simulink model "VSI_o_loop_Gvd"  (Simulink 7.8)
settings: Solver=ode23t  StartTime=0.0  StopTime=0.5  MaxStep=25e-6  RelTol=1e-4  AbsTol=1e-5
values from neighbouring files (symbols this model uses):
  C = 21.308e-6    (= 2.1308e-05)    [Current_Loop_Design.m]    (also in VSI_Controller_Design.m = 3.13e-05; VSI_TFs_i_loop.m = 2.2e-05; VSI_TFs_o_loop.m = 4.13e-05; VSI_TFs_v_loop.m = 4.1308e-05)
  Dd = -(omega*L*Voq-Rac*Vod-Rl*Vod+Rl*omega*C*Voq*Rac+omega^2*L*C*Vod*Rac)/(Rac*Vdc)    [Current_Loop_Design.m]    (also in ZVSI_il_tf_cal_sim_comp_frd_model_v1.m = Dd(length(Dd)-10); ZVSI_ol_tf_cal_sim_comp_frd_model_v1.m = 0.295957004555; ZVSI_vil_tf_cal_frd_model_Monte_Carlo.m; ZVSI_vil_tf_cal_sim_comp_frd_model_v1.m = Dd(length(Dd)-10))
  Dq = -(-Rl*Voq-Rac*Voq-omega*L*Vod+omega^2*L*C*Voq*Rac-Rl*omega*C*Vod*Rac)/(Rac*Vdc)    [Current_Loop_Design.m]    (also in ZVSI_il_tf_cal_sim_comp_frd_model_v1.m = Dq(length(Dq)-10); ZVSI_ol_tf_cal_sim_comp_frd_model_v1.m = 0.0618083618596; ZVSI_vil_tf_cal_frd_model_Monte_Carlo.m; ZVSI_vil_tf_cal_sim_comp_frd_model_v1.m = Dq(length(Dq)-10))
  L = (0.75879e-3)/(2/3)    (= 0.001138185)    [Current_Loop_Design.m]    (also in VSI_Controller_Design.m = 0.0011; VSI_TFs_i_loop.m = 0.0012; VSI_TFs_o_loop.m = 0.0011; VSI_TFs_v_loop.m = 0.0011)
  RL = 80e-3    (= 0.08)    [Current_Loop_Design.m]    (also in ZVSI_il_tf_cal_sim_comp_frd_model_v1.m = 0.15; ZVSI_ol_tf_cal_sim_comp_frd_model_v1.m = 1.5e-05; ZVSI_vil_tf_cal_frd_model_Monte_Carlo.m = 0.13; ZVSI_vil_tf_cal_sim_comp_frd_model_v1.m = 0.13)
  Vdc = 270    [Current_Loop_Design.m]    (also in VSI_Controller_Design.m; VSI_TFs_i_loop.m; VSI_TFs_o_loop.m; VSI_TFs_v_loop.m)
  w = 2*pi*fline    (= 2513.27412287)    [Current_Loop_Design.m]    (also in ZVSI_il_tf_cal_sim_comp_frd_model_v1.m = 15791.3670417; ZVSI_ol_tf_cal_sim_comp_frd_model_v1.m = 15791.3670417; ZVSI_vil_tf_cal_frd_model_Monte_Carlo.m = 15791.3670417; ZVSI_vil_tf_cal_sim_comp_frd_model_v1.m = 15791.3670417)
libraries: powerlib x20
settings Model: Creator=marko  LastModifiedBy=wenbo  BufferReuse=off
settings OptimizationCC: BlockReduction=off  InlineParams=on  BufferReuse=off
settings DebuggingCC: AlgebraicLoopMsg=none  SolverPrmCheckMsg=none  FcnCallInpInsideContextMsg=Use local settings  UnconnectedInputMsg=none  UnconnectedOutputMsg=none  UnconnectedLineMsg=none  StrictBusMsg=Warning

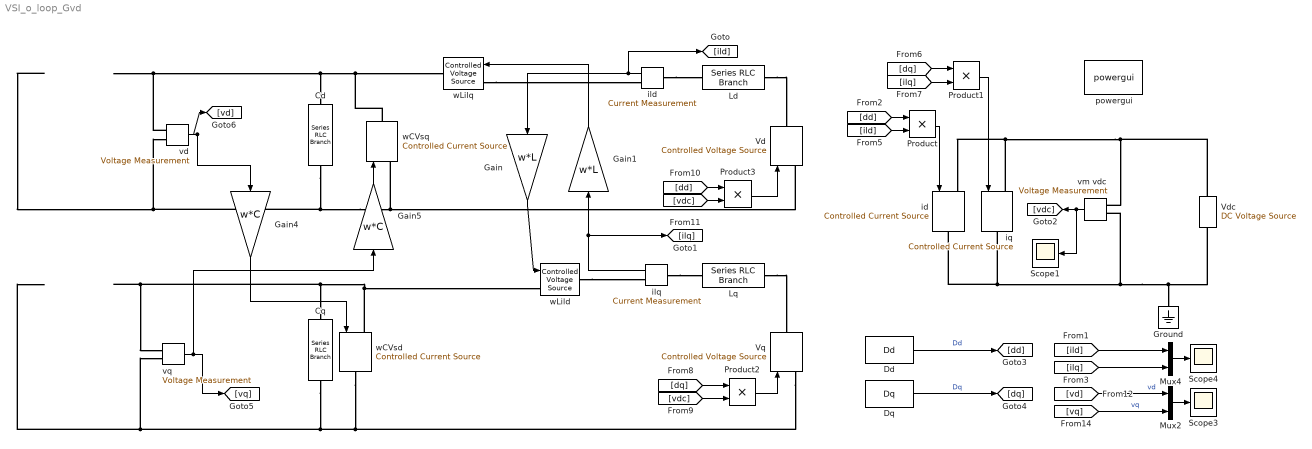
== system VSI_o_loop_Gvd ==
  Cd : powerlib/Elements/Series RLC Branch  LConnTagsString=__new0  RConnTagsString=__new0  BranchType=C  Resistance=1  Inductance=1e-3  SetiL0=off  InitialCurrent=0  Capacitance=C  Setx0=off  InitialVoltage=0  Measurements=None
  Cq : powerlib/Elements/Series RLC Branch  LConnTagsString=__new0  RConnTagsString=__new0  BranchType=C  Resistance=1  Inductance=1e-3  SetiL0=off  InitialCurrent=0  Capacitance=C  Setx0=off  InitialVoltage=0  Measurements=None
  Dd : Constant  Value=Dd
  Dq : Constant  Value=Dq
  Gain : Gain  Gain=w*L
  Gain1 : Gain  Gain=w*L
  Gain4 : Gain  Gain=w*C
  Gain5 : Gain  Gain=w*C
  Ground : powerlib/Elements/Ground  LConnTagsString=a
  Ld : powerlib/Elements/Series RLC Branch  LConnTagsString=__new0  RConnTagsString=__new0  BranchType=RL  Resistance=RL  Inductance=L  SetiL0=off  InitialCurrent=0  Capacitance=1e-6  Setx0=off  InitialVoltage=0  Measurements=None
  Lq : powerlib/Elements/Series RLC Branch  LConnTagsString=__new0  RConnTagsString=__new0  BranchType=RL  Resistance=RL  Inductance=L  SetiL0=off  InitialCurrent=0  Capacitance=1e-6  Setx0=off  InitialVoltage=0  Measurements=None
  Mux2 : Mux  Inputs=2
  Mux4 : Mux  Inputs=2
  Product{,1..3} (4 alike) : Product  RndMeth=Zero
  Scope1 : Scope
      settings: YMin=270  YMax=270  SaveName=ildq_matlab  DataFormat=Array
  Scope3 : Scope
      settings: YMin=-0.25  YMax=5.25  SaveName=ildq_matlab2  DataFormat=Array
  Scope4 : Scope
      settings: YMin=-0.25  YMax=5.25  SaveName=ildq_matlab1  DataFormat=Array
  Vd : powerlib/Electrical Sources/Controlled Voltage Source  Initialize=on  Source_Type=DC  Amplitude=0  Phase=0  Frequency=0  Measurements=None
  Vdc : powerlib/Electrical Sources/DC Voltage Source  Amplitude=Vdc  Measurements=None
  Vq : powerlib/Electrical Sources/Controlled Voltage Source  Initialize=on  Source_Type=DC  Amplitude=0  Phase=0  Frequency=0  Measurements=None
  id : powerlib/Electrical Sources/Controlled Current Source  Initialize=on  Source_Type=DC  Amplitude=0  Phase=0  Frequency=0  Measurements=None
  ild : powerlib/Measurements/Current Measurement  PhasorSimulation=off  OutputType=Complex  PSBequivalent=0
  ilq : powerlib/Measurements/Current Measurement  PhasorSimulation=off  OutputType=Complex  PSBequivalent=0
  iq : powerlib/Electrical Sources/Controlled Current Source  Initialize=on  Source_Type=DC  Amplitude=0  Phase=0  Frequency=0  Measurements=None
  powergui : powerlib/powergui  Priority=1  SimulationMode=Continuous  SolverType=Tustin  SampleTime=50e-6  frequency=60  SPID=off  DisableSnubberDevices=off  DisableRonSwitches=off  DisableVfSwitches=off  SwTol=0  Interpol=off  DisplayEquations=off  FunctionMessages=off  frequencyindice=0  Pbase=100e6  ErrMax=1e-4  Iterations=50  UnitsV=kV  UnitsW=MW  echomessages=off  HookPort=off  EnableUseOfTLC=off  x0status=blocks  RestoreLinks=warning  ResistiveCurrentMeasurement=off  Frange=[0:2:500]  Ylog=off  Xlog=on  ShowGrid=off  save=off  variable=ZData  ZoomFFT=on  StartTime=0.0  cycles=1  DisplayStyle=1  fundamental=60  FreqAxis=off  MaxFrequency=1000  frequencyindicesteady=1  RmsSteady=1  display=off  Ts=0  methode=off
  vd : powerlib/Measurements/Voltage Measurement  PhasorSimulation=off  OutputType=Complex  PSBequivalent=0
  vm vdc : powerlib/Measurements/Voltage Measurement  PhasorSimulation=off  OutputType=Complex  PSBequivalent=0
  vq : powerlib/Measurements/Voltage Measurement  PhasorSimulation=off  OutputType=Complex  PSBequivalent=0
  wCVsd : powerlib/Electrical Sources/Controlled Current Source  Initialize=on  Source_Type=DC  Amplitude=0  Phase=0  Frequency=0  Measurements=None
  wCVsq : powerlib/Electrical Sources/Controlled Current Source  Initialize=on  Source_Type=DC  Amplitude=0  Phase=0  Frequency=0  Measurements=None
  wLild : powerlib/Electrical Sources/Controlled Voltage Source  Initialize=on  Source_Type=DC  Amplitude=0  Phase=0  Frequency=0  Measurements=None
  wLilq : powerlib/Electrical Sources/Controlled Voltage Source  Initialize=on  Source_Type=DC  Amplitude=0  Phase=0  Frequency=0  Measurements=None
  wires:
  Product/1 -> id/1
  [dd] -> Product/1
  [ild] -> Product/2
  Product1/1 -> iq/1
  [dq] -> Product1/1
  [ilq] -> Product1/2
  [dq] -> Product2/1
  [vdc] -> Product2/2
  Product2/1 -> Vq/1
  [dd] -> Product3/1
  [vdc] -> Product3/2
  Product3/1 -> Vd/1
  vd/1 -> Gain4/1, [vd]
  vq/1 -> Gain5/1, [vq]
  vm vdc/1 -> [vdc], Scope1/1
  ilq/1 -> Gain1/1, [ilq]
  Gain1/1 -> wLilq/1
  ild/1 -> Gain/1, [ild]
  Gain/1 -> wLild/1
  Gain4/1 -> wCVsd/1
  Gain5/1 -> wCVsq/1
  Dd/1 -> [dd]  "Dd"
  Dq/1 -> [dq]  "Dq"
  [ild] -> Mux4/1
  [ilq] -> Mux4/2
  Mux4/1 -> Scope4/1
  [vd] -> Mux2/1  "vd"
  [vq] -> Mux2/2  "vq"
  Mux2/1 -> Scope3/1
  connections:
  Vq/LConn1 -- wCVsd/RConn1 -- Cq/RConn1 -- vq/LConn2
  iq/RConn1 -- id/RConn1 -- vm vdc/LConn2 -- Ground/LConn1 -- Vdc/LConn1
  Cq/LConn1 -- wCVsd/LConn1 -- wLild/LConn1 -- vq/LConn1
  wLilq/LConn1 -- ild/RConn1
  wLild/RConn1 -- ilq/RConn1
  ilq/LConn1 -- Lq/LConn1
  ild/LConn1 -- Ld/LConn1
  Ld/RConn1 -- Vd/RConn1
  Lq/RConn1 -- Vq/RConn1
  Vdc/RConn1 -- iq/LConn1 -- id/LConn1 -- vm vdc/LConn1
  wCVsq/RConn1 -- wLilq/RConn1 -- Cd/LConn1 -- vd/LConn1
  Vd/LConn1 -- wCVsq/LConn1 -- Cd/RConn1 -- vd/LConn2
